simulink model "dynamic_model_dab_battery"  (R2022b)
settings: Solver=VariableStepAuto  StartTime=0.0  StopTime=5e-2  RelTol=1e-3
undefined symbols (not defined in the file): Ion, Lithium
libraries: spsMosfetLib x8, spsSeriesRLCBranchLib x6, spsEdgeDetectorLib x4, spsCurrentMeasurementLib x3, spsDiscreteVariableTimeDelayLib x2, spsBatteryLib x1, spsDCVoltageSourceLib x1, spsMultimeterLib x1, spsStairGeneratorLib x1, slpidlib x1, spsLinearTransformerLib x1, spsVoltageMeasurementLib x1
settings Model: Creator=srikr  LastModifiedBy=srikri

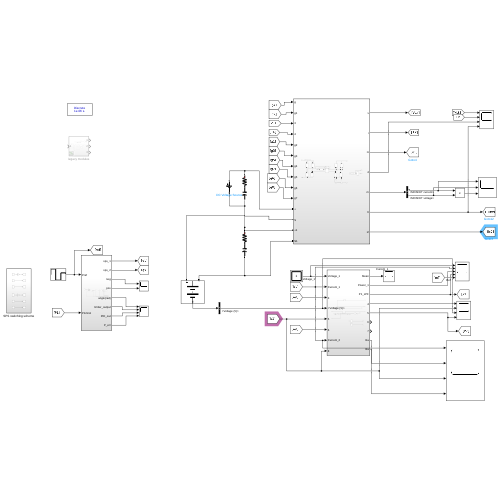
[thumbnail: Simulink's stored preview of the top-level diagram]
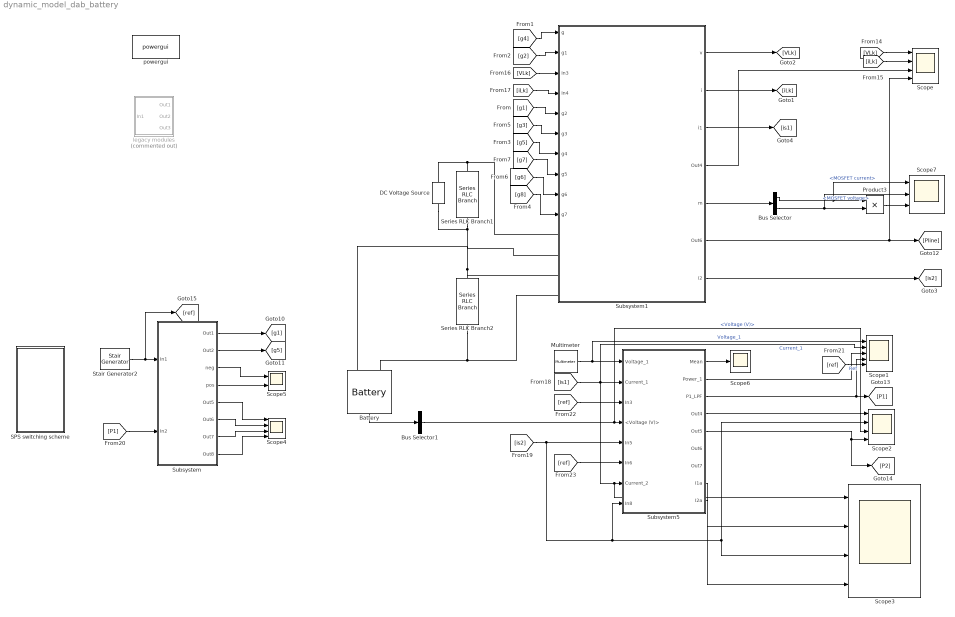
== system dynamic_model_dab_battery ==
  Battery : spsBatteryLib/Battery  BatType=Lithium-Ion  ShowTempParam=off  ThermalPreset=no  ShowAgeParam=off  NomV=96  NomQ=150  SOC=100  Batt_Tr=30  PresetModel=on  MaxQ=150  MinV=72  FullV=111.7428  Dis_rate=65.2174  R=0.0064  Normal_OP=135.6522  expZone="[103.717      7.369565]"  current=[6.5 13 32.5]  Units=Time  Tci=20  NomT=20  T2=-30  MaxQ2=4.8  FullV2=7.1  Normal_OP2=5.655  expZone2="[6.58           1]"  Rca=0.6  ti=2000  Dp=0  Neq0=0  Tsim=1e6  Ta1=25  Qeol=5.4*0.9  Reol=0.013333*1.2  Char_age=[2.3478, 3]  Dis_age=[2.3478, 10]  N1=1500  N2=10500  N3=1000  N4=1400  Ta2=45  N5=950
  Bus Selector : BusSelector  OutputSignals=MOSFET current,MOSFET voltage
  Bus Selector1 : BusSelector  OutputSignals=Voltage (V)
  DC Voltage Source : spsDCVoltageSourceLib/DC Voltage Source  Amplitude=120  Measurements=Voltage
  Multimeter : spsMultimeterLib/Multimeter  L=10  sel=4  yselected={}  Gain=1  OutputType=Complex  PlotAtSimulationStop=off  PhasorSimulation=off
  Product3 : Product
  SPS switching scheme : Subsystem
  Scope{,2..4} (4 alike) : Scope  NumInputPorts=4
  Scope1 : Scope  NumInputPorts=5
  Scope5 : Scope  NumInputPorts=2
  Scope6 : Scope
  Scope7 : Scope  NumInputPorts=3
  Series RLC Branch1 : spsSeriesRLCBranchLib/Series RLC Branch  LConnTagsString=__new0  RConnTagsString=__new0  BranchType=RC  Resistance=1e-9  Inductance=1e-3  SetiL0=off  InitialCurrent=0  Capacitance=1000e-6  Setx0=off  InitialVoltage=0  Measurements=None
  Series RLC Branch2 : spsSeriesRLCBranchLib/Series RLC Branch  LConnTagsString=__new0  RConnTagsString=__new0  BranchType=RC  Resistance=1e-9  Inductance=1e-3  SetiL0=off  InitialCurrent=0  Capacitance=1000e-6  Setx0=off  InitialVoltage=0  Measurements=None
  Stair Generator2 : spsStairGeneratorLib/Stair Generator  t=[0:.25:1]*4e-2  e=[0e3,3.5e3,-3.5e3,1e3,0.5e3]  Ts=0
  Subsystem : Subsystem
  Subsystem1 : Subsystem
  Subsystem5 : Subsystem
  legacy modules : Subsystem  Commented=on
  powergui : spspowerguiLib/powergui  Priority=1  SimulationMode=Discrete  SampleTime=1e-6  frequency=60  Iterations=50  frequencyindice=0  Pbase=100e6  ErrMax=1e-4  UnitsV=kV  UnitsW=MW  buscounter=0  FunctionMessages=off  echomessages=off  EnableUseOfTLC=off  CurrentSourceSwitches=off  DisableSnubberDevices=off  DisableRonSwitches=off  DisableVfSwitches=off  DisplayEquations=off  AutomaticDiscreteSolvers=off  SolverType=Tustin/Backward Euler (TBE)  Interpol=off  ExternalGateDelay=off  methode=off  Ts=100  x0status=blocks  SPID=on  SwTol=0  HookPort=off  NonlinearTolerance=1e-4  nMaxIteration=100  ContinueOnMaxIteration=off  RestoreLinks=warning  ResistiveCurrentMeasurement=off  Frange=[0:2:500]  Ylog=off  Xlog=on  ShowGrid=off  save=off  variable=ZData  structure=0  ZoomFFT=off  StartTime=0.0  cycles=1  DisplayStyle=1  fundamental=60  FreqAxis=off  MaxFrequency=1000  frequencyindicesteady=1  RmsSteady=1  display=off
  wires:
  [VLk] -> Scope/1
  [iLk] -> Scope/2
  Multimeter/1 -> Scope1/1, Subsystem5/1(Voltage_1)  "Voltage_1"
  [is1] -> Scope1/2, Scope3/1, Subsystem5/7(Current_2), Subsystem5/2(Current_1)  "Current_1"
  [is2] -> Scope2/2, Scope3/3, Subsystem5/8(In8), Subsystem5/5(In5)
  Bus Selector1/1 -> Scope2/1, Subsystem5/4(<Voltage (V)>)  "<Voltage (V)>"
  Stair Generator2/1 -> [ref], Subsystem/1(In1)
  Bus Selector/1 -> Scope7/1, Product3/1  "<MOSFET current>"
  Bus Selector/2 -> Scope7/2, Product3/2  "<MOSFET voltage>"
  Product3/1 -> Scope7/3
  [ref] -> Scope1/5  "Ref"
  Battery/1 -> Bus Selector1/1
  [P1] -> Subsystem/2(In2)
  Subsystem/1(Out1) -> [g1]
  Subsystem/2(Out2) -> [g5]
  Subsystem/3(neg) -> Scope5/1
  Subsystem/4(pos) -> Scope5/2
  Subsystem/5(Out5) -> Scope4/1
  Subsystem/6(Out6) -> Scope4/2
  Subsystem/7(Out7) -> Scope4/3
  Subsystem/8(Out8) -> Scope4/4
  Subsystem5/5(Out5) -> [P2], Scope2/4
  Subsystem5/3(P1_LPF) -> [P1], Scope1/4
  [ref] -> Subsystem5/3(In3)
  [ref] -> Subsystem5/6(In6)
  Subsystem5/1(Mean) -> Scope6/1
  Subsystem5/2(Power_1) -> Scope1/3
  Subsystem5/4(Out4) -> Scope2/3
  Subsystem5/8(I1a) -> Scope3/2
  Subsystem5/9(I2a) -> Scope3/4
  Subsystem1/6(Out6) -> [Pline], Scope/4
  [g4] -> Subsystem1/1(g)
  [g2] -> Subsystem1/2(g1)
  [VLk] -> Subsystem1/3(In3)
  [iLk] -> Subsystem1/4(In4)
  [g1] -> Subsystem1/5(g2)
  [g3] -> Subsystem1/6(g3)
  [g5] -> Subsystem1/7(g4)
  [g7] -> Subsystem1/8(g5)
  [g6] -> Subsystem1/9(g6)
  [g8] -> Subsystem1/10(g7)
  Subsystem1/1(v) -> [VLk]
  Subsystem1/2(i) -> [iLk]
  Subsystem1/3(i1) -> [is1]
  Subsystem1/4(Out4) -> Scope/3
  Subsystem1/5(m) -> Bus Selector/1
  Subsystem1/7(i2) -> [is2]
  connections:
  Series RLC Branch1/RConn1 -- DC Voltage Source/LConn1 -- Subsystem1/LConn2
  Series RLC Branch2/RConn1 -- Battery/LConn2 -- Subsystem1/LConn4
  Series RLC Branch2/LConn1 -- Battery/LConn1 -- Subsystem1/LConn3
  DC Voltage Source/RConn1 -- Subsystem1/LConn1 -- Series RLC Branch1/LConn1

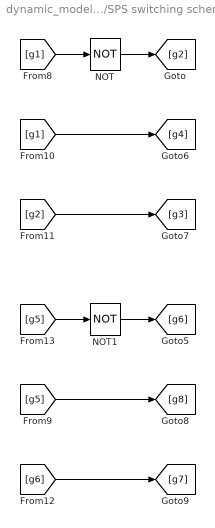
== system dynamic_model_dab_battery/SPS switching scheme ==
  NOT : Logic  Operator=NOT  IconShape=distinctive  AllPortsSameDT=off  OutDataTypeStr=boolean
  NOT1 : Logic  Operator=NOT  IconShape=distinctive  AllPortsSameDT=off  OutDataTypeStr=boolean
  wires:
  [g1] -> [g4]
  [g2] -> [g3]
  [g5] -> NOT1/1
  [g6] -> [g7]
  NOT1/1 -> [g6]
  [g5] -> [g8]
  NOT/1 -> [g2]
  [g1] -> NOT/1

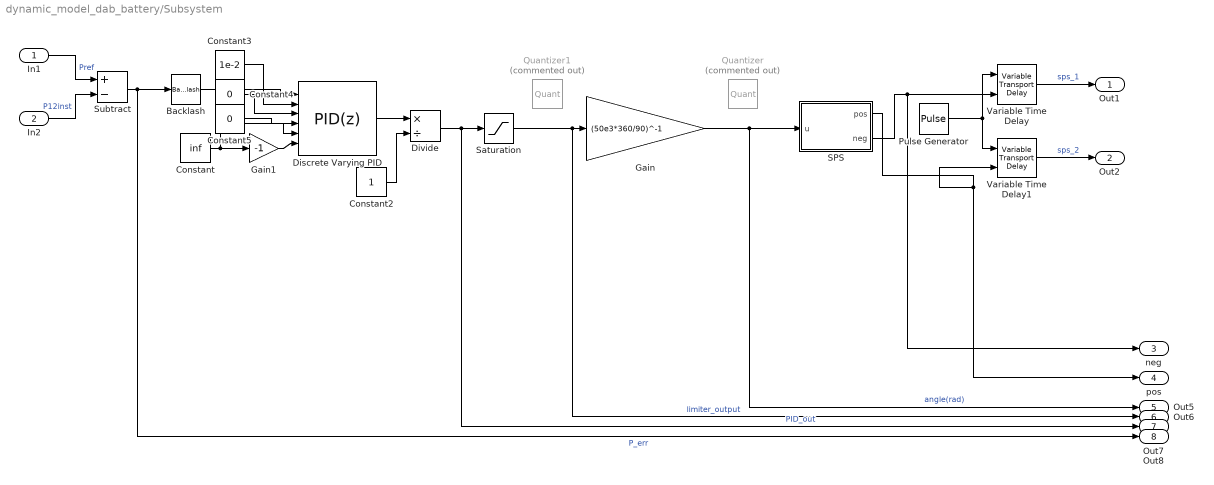
== system dynamic_model_dab_battery/Subsystem ==
  In1 : Inport
  In2 : Inport  Port=2
  Backlash : Backlash  BacklashWidth=0
  Constant : Constant  Value=inf
  Constant2 : Constant
  Constant3 : Constant  Value=1e-2
  Constant4 : Constant  Value=0
  Constant5 : Constant  Value=0
  Discrete Varying PID : slpidlib/PID Controller  Controller=PID  Form=Parallel  TimeDomain=Discrete-time  UseExternalTs=off  SampleTime=-1  IntegratorMethod=Forward Euler  FilterMethod=Forward Euler  ControllerParametersSource=external  P=1  I=1  UseKiTs=off  D=0  N=100  UseFilter=off  TunerSelectOption=Transfer Function Based (PID Tuner App)  InitialConditionSource=internal  InitialConditionForIntegrator=0  InitialConditionForFilter=0  DifferentiatorICPrevScaledInput=0  ExternalReset=none  TrackingMode=off  Kt=1  LimitOutput=on  SatLimitsSource=external  UpperSaturationLimit=inf  LowerSaturationLimit=-inf  LinearizeAsGain=on  AntiWindupMode=none  Kb=1  LimitIntegrator=off  UpperIntegratorSaturationLimit=inf  LowerIntegratorSaturationLimit=-inf  POutMin=[]  POutMax=[]  IOutMin=[]  IOutMax=[]  DOutMin=[]  DOutMax=[]  NOutMin=[]  NOutMax=[]  SumOutMin=[]  SumOutMax=[]  SaturationOutMin=[]  SaturationOutMax=[]  PParamMin=[]  PParamMax=[]  IParamMin=[]  IParamMax=[]  DParamMin=[]  DParamMax=[]  NParamMin=[]  NParamMax=[]  KbParamMin=[]  KbParamMax=[]  KtParamMin=[]  KtParamMax=[]  KbOutMin=[]  KbOutMax=[]  KtOutMin=[]  KtOutMax=[]  IntegratorOutMin=[]  IntegratorOutMax=[]  FilterOutMin=[]  FilterOutMax=[]  SumI1OutMin=[]  SumI1OutMax=[]  SumI2OutMin=[]  SumI2OutMax=[]  SumI3OutMin=[]  SumI3OutMax=[]  SumI4OutMin=[]  SumI4OutMax=[]  SumDOutMin=[]  SumDOutMax=[]  DifferentiatorOutMin=[]  DifferentiatorOutMax=[]  FilterDiffOutCoefMin=[]  FilterDiffOutCoefMax=[]  ReciprocalOutMin=[]  ReciprocalOutMax=[]  SumDenOutMin=[]  SumDenOutMax=[]  SumNumOutMin=[]  SumNumOutMax=[]  DivideOutMin=[]  DivideOutMax=[]  UdiffTsProdOutMin=[]  UdiffTsProdOutMax=[]  NTsProdOutMin=[]  NTsProdOutMax=[]  UintegralTsProdOutMin=[]  UintegralTsProdOutMax=[]  UngainTsProdOutMin=[]  UngainTsProdOutMax=[]  ClampingZeroOutDataTypeStr=Inherit: Inherit via back propagation  ClampingZeroOutMin=[]  ClampingZeroOutMax=[]  FilterDenConstantOutDataTypeStr=Inherit: Inherit via back propagation  FilterDenConstantOutMin=[]  FilterDenConstantOutMax=[]  PCopyOutDataTypeStr=Inherit: Inherit via back propagation  PCopyOutMin=[]  PCopyOutMax=[]  NCopyOutDataTypeStr=Inherit: Inherit via back propagation  NCopyOutMin=[]  NCopyOutMax=[]  IntegratorContinuousStateAttributes=''  IntegratorStateMustResolveToSignalObject=off  IntegratorRTWStateStorageClass=Auto  FilterContinuousStateAttributes=''  FilterStateMustResolveToSignalObject=off  FilterRTWStateStorageClass=Auto  ParallelPVariant=ExternalParameters  IdealPVariant=Disabled  IVariant=ExternalParameters  DVariant=ExternalParameters  IntegratorVariant=Discrete  SatVariant=External  AWVariant=Passthrough  PCopyVariant=Disabled  TRVariant=Disabled  FdbkBlocksVariant=Forward  IdealPFdbkVariant=Disabled  SatFdbkVariant=Disabled  DerivativeFilterVariant=Differentiator  NVariant=Passthrough  NCopyVariant=Disabled_SignalSpec  FilterICVariant=InternalICsDifferentiator  IntegratorICVariant=InternalICs  ExternalResetVariant=Disabled  TRSumVariant=Passthrough  SumFdbkVariant=Disabled  SumVariant=Sum_PID  TsampFilterVariant=InternalTs  TsampNgainVariant=Passthrough  TsampIntegralVariant=Passthrough  ExternalSaturationOutDataTypeStr=Inherit: Same as second input
      settings: LibrarySourceBlock=cstblocks/Linear Parameter Varying/Discrete Varying PID
  Divide : Product  Inputs=*/
  Gain : Gain  Gain=(50e3*360/90)^-1
  Gain1 : Gain  Gain=-1
  Pulse Generator : DiscretePulseGenerator  PulseType=Time based  Period=1/50e3  PulseWidth=50
  Quantizer : Quantizer  Commented=on  QuantizationInterval=1e-5
  Quantizer1 : Quantizer  Commented=on  QuantizationInterval=1e-2
  SPS : MATLAB Function  TreatAsAtomicUnit=on
  Saturation : Saturate  UpperLimit=1  LowerLimit=-1
  Subtract : Sum  Inputs=+-
  Variable Time Delay : VariableTransportDelay  MaximumDelay=10
  Variable Time Delay1 : VariableTransportDelay  MaximumDelay=10
  Out1 : Outport
  Out2 : Outport  Port=2
  neg : Outport  Port=3
  pos : Outport  Port=4
  Out5 : Outport  Port=5
  Out6 : Outport  Port=6
  Out7 : Outport  Port=7
  Out8 : Outport  Port=8
  wires:
  Backlash/1 -> Discrete Varying PID/1
  Constant2/1 -> Divide/2
  Constant4/1 -> Discrete Varying PID/3
  In1/1 -> Subtract/1  "Pref"
  Variable Time Delay/1 -> Out1/1  "sps_1"
  Saturation/1 -> Out6/1, Gain/1  "limiter_output"
  SPS/1(pos) -> pos/1, Variable Time Delay1/2
  SPS/2(neg) -> neg/1, Variable Time Delay/2
  Variable Time Delay1/1 -> Out2/1  "sps_2"
  In2/1 -> Subtract/2  "P12inst"
  Constant/1 -> Discrete Varying PID/5, Gain1/1
  Constant5/1 -> Discrete Varying PID/4
  Pulse Generator/1 -> Variable Time Delay1/1, Variable Time Delay/1
  Constant3/1 -> Discrete Varying PID/2
  Divide/1 -> Out7/1, Saturation/1  "PID_out"
  Discrete Varying PID/1 -> Divide/1
  Subtract/1 -> Out8/1, Backlash/1  "P_err"
  Gain1/1 -> Discrete Varying PID/6
  Gain/1 -> Out5/1, SPS/1(u)  "angle(rad)"

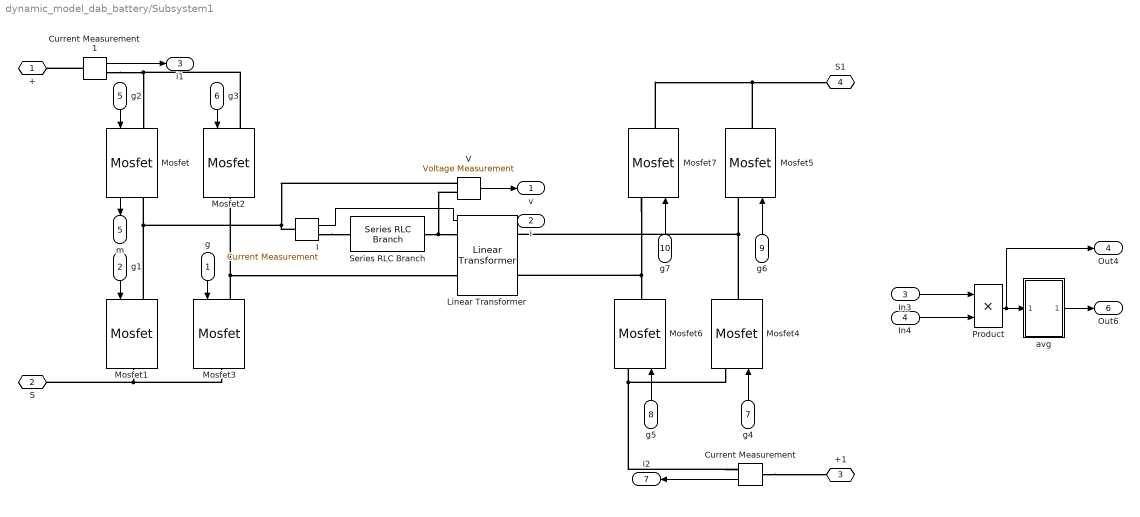
== system dynamic_model_dab_battery/Subsystem1 ==
  g : Inport
  g1 : Inport  Port=2
  In3 : Inport  Port=3
  In4 : Inport  Port=4
  g2 : Inport  Port=5
  g3 : Inport  Port=6
  g4 : Inport  Port=7
  g5 : Inport  Port=8
  g6 : Inport  Port=9
  g7 : Inport  Port=10
  Current Measurement : spsCurrentMeasurementLib/Current Measurement  PhasorSimulation=off  OutputType=Complex  PSBequivalent=0
  Current Measurement1 : spsCurrentMeasurementLib/Current Measurement  PhasorSimulation=off  OutputType=Complex  PSBequivalent=0
  I : spsCurrentMeasurementLib/Current Measurement  PhasorSimulation=off  OutputType=Complex  PSBequivalent=0
  Linear Transformer : spsLinearTransformerLib/Linear Transformer  UNITS=SI  NominalPower=[ 3.5e3 50e3 ]  winding1=[120 0 0]  winding2=[96 0 0]  ThreeWindings=off  winding3=[3.15e+05 0.7938 0.084225]  RmLm=[10e6 2e-3]  Measurements=All voltages and currents  DataType=on
  Mosfet : spsMosfetLib/Mosfet  Ron=0.1  Lon=0  Rd=0.01  Vfd=0  IC=0  Rs=1e6  Cs=inf  Measurements=on
  Mosfet1 : spsMosfetLib/Mosfet  Ron=0.1  Lon=0  Rd=0.01  Vfd=0  IC=0  Rs=inf  Cs=inf  Measurements=off
  Mosfet{2..7} (6 alike) : spsMosfetLib/Mosfet  Ron=0.1  Lon=0  Rd=0.01  Vfd=0  IC=0  Rs=1e6  Cs=inf  Measurements=off
  Product : Product
  Series RLC Branch : spsSeriesRLCBranchLib/Series RLC Branch  LConnTagsString=__new0  RConnTagsString=__new0  BranchType=L  Resistance=1  Inductance=15e-6  SetiL0=off  InitialCurrent=0  Capacitance=1e-6  Setx0=off  InitialVoltage=0  Measurements=Branch voltage and current
  V : spsVoltageMeasurementLib/Voltage Measurement  PhasorSimulation=off  OutputType=Complex  PSBequivalent=0
  avg : Subsystem
  + : PMIOPort  Side=Left
  S : PMIOPort  Port=2  Side=Left
  +1 : PMIOPort  Port=3  Side=Left
  S1 : PMIOPort  Port=4  Side=Left
  v : Outport
  i : Outport  Port=2
  i1 : Outport  Port=3
  Out4 : Outport  Port=4
  m : Outport  Port=5
  Out6 : Outport  Port=6
  i2 : Outport  Port=7
  wires:
  V/1 -> v/1
  g5/1 -> Mosfet6/1
  In3/1 -> Product/1
  g6/1 -> Mosfet5/1
  In4/1 -> Product/2
  Mosfet/1 -> m/1
  g2/1 -> Mosfet/1
  g4/1 -> Mosfet4/1
  I/1 -> i/1
  Current Measurement1/1 -> i1/1
  Current Measurement/1 -> i2/1
  g1/1 -> Mosfet1/1
  g/1 -> Mosfet3/1
  avg/1(Out1) -> Out6/1
  g3/1 -> Mosfet2/1
  g7/1 -> Mosfet7/1
  Product/1 -> Out4/1, avg/1(In1)
  connections:
  Mosfet7/LConn1 -- Mosfet6/RConn1 -- Linear Transformer/RConn2
  Current Measurement1/RConn1 -- Mosfet/LConn1 -- Mosfet2/LConn1
  Series RLC Branch/RConn1 -- V/LConn2 -- Linear Transformer/LConn1
  Current Measurement/LConn1 -- +1/RConn1
  Current Measurement/RConn1 -- Mosfet4/LConn1 -- Mosfet6/LConn1
  Mosfet4/RConn1 -- Mosfet5/LConn1 -- Linear Transformer/RConn1
  Current Measurement1/LConn1 -- +/RConn1
  Mosfet3/RConn1 -- S/RConn1 -- Mosfet1/RConn1
  I/LConn1 -- V/LConn1 -- Mosfet1/LConn1 -- Mosfet/RConn1
  I/RConn1 -- Series RLC Branch/LConn1
  Mosfet7/RConn1 -- Mosfet5/RConn1 -- S1/RConn1
  Mosfet3/LConn1 -- Linear Transformer/LConn2 -- Mosfet2/RConn1

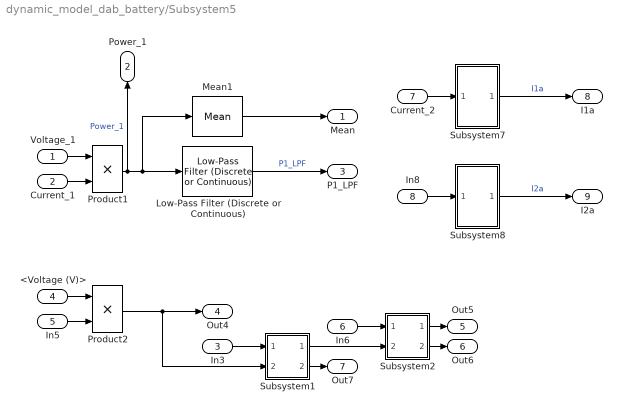
== system dynamic_model_dab_battery/Subsystem5 ==
  Voltage_1 : Inport
  Current_1 : Inport  Port=2
  In3 : Inport  Port=3
  <Voltage (V)> : Inport  Port=4
  In5 : Inport  Port=5
  In6 : Inport  Port=6
  Current_2 : Inport  Port=7
  In8 : Inport  Port=8
  Low-Pass Filter (Discrete or Continuous) : eeGeneralControl/Low-Pass Filter (Discrete or Continuous)  K=1  T=1e-3  B=inf  A=-inf  init_option=Specify as parameter  x0=0  Ts=-1
  Mean1 : spsMeanLib/Mean  Freq=25e3  Vinit=0  Ts=0
  Product1 : Product
  Product2 : Product
  Subsystem1 : Subsystem
  Subsystem2 : Subsystem
  Subsystem7 : Subsystem
  Subsystem8 : Subsystem
  Mean : Outport
  Power_1 : Outport  Port=2
  P1_LPF : Outport  Port=3
  Out4 : Outport  Port=4
  Out5 : Outport  Port=5
  Out6 : Outport  Port=6
  Out7 : Outport  Port=7
  I1a : Outport  Port=8
  I2a : Outport  Port=9
  wires:
  Current_2/1 -> Subsystem7/1(In1)
  Subsystem7/1(Out1) -> I1a/1  "I1a"
  Subsystem8/1(Out1) -> I2a/1  "I2a"
  Current_1/1 -> Product1/2
  Low-Pass Filter (Discrete or Continuous)/1 -> P1_LPF/1  "P1_LPF"
  In8/1 -> Subsystem8/1(In1)
  Mean1/1 -> Mean/1
  Product2/1 -> Out4/1, Subsystem1/2(In2)
  Product1/1 -> Low-Pass Filter (Discrete or Continuous)/1, Mean1/1, Power_1/1  "Power_1"
  In6/1 -> Subsystem2/1(In1)
  <Voltage (V)>/1 -> Product2/1
  In3/1 -> Subsystem1/1(In1)
  Subsystem2/2(Out2) -> Out6/1
  Voltage_1/1 -> Product1/1
  In5/1 -> Product2/2
  Subsystem1/1(Out1) -> Subsystem2/2(In2)
  Subsystem2/1(Out1) -> Out5/1
  Subsystem1/2(Out2) -> Out7/1

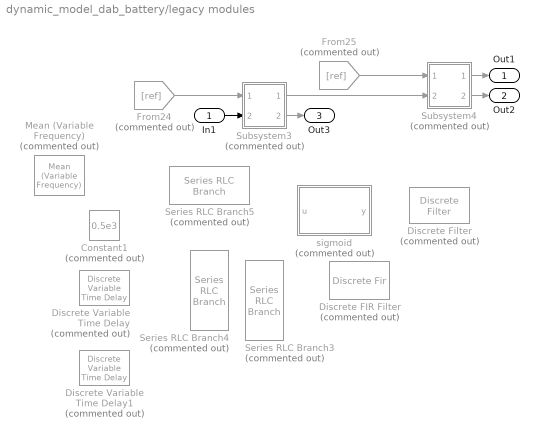
== system dynamic_model_dab_battery/legacy modules ==
  In1 : Inport
  Constant1 : Constant  Commented=on  Value=0.5e3
  Discrete FIR Filter : DiscreteFir  Commented=on
  Discrete Filter : DiscreteFilter  Commented=on
  Discrete Variable Time Delay : spsDiscreteVariableTimeDelayLib/Discrete Variable Time Delay  Commented=on  MaxDelay=1  InitialValue=0  Ts=1e-4  DFT=on
      settings: LibrarySourceBlock=|
      | sps_lib/Control/Discrete Variable
      | Time Delay
  Discrete Variable Time Delay1 : spsDiscreteVariableTimeDelayLib/Discrete Variable Time Delay  Commented=on  MaxDelay=1  InitialValue=0  Ts=1e-4  DFT=on
      settings: LibrarySourceBlock=|
      | sps_lib/Control/Discrete Variable
      | Time Delay
  From24 : From  Commented=on  GotoTag=ref
  From25 : From  Commented=on  GotoTag=ref
  Mean (Variable Frequency) : spsMeanVariableFrequencyLib/Mean (Variable Frequency)  Commented=on  Finit=60  Fmin=45  Vinit=0  Ts=0
      settings: LibrarySourceBlock=|
      | sps_lib/Sensors and Measurements/Mean
      | (Variable Frequency)
  Series RLC Branch3 : spsSeriesRLCBranchLib/Series RLC Branch  Commented=on  LConnTagsString=__new0  RConnTagsString=__new0  BranchType=L  Resistance=1  Inductance=1e-6/(1.25^2)  SetiL0=off  InitialCurrent=0  Capacitance=1e-6  Setx0=off  InitialVoltage=0  Measurements=Branch voltage and current
  Series RLC Branch4 : spsSeriesRLCBranchLib/Series RLC Branch  Commented=on  LConnTagsString=__new0  RConnTagsString=__new0  BranchType=C  Resistance=1  Inductance=14e-6  SetiL0=off  InitialCurrent=0  Capacitance=10e-6*(1.25^2)  Setx0=off  InitialVoltage=0  Measurements=Branch voltage and current
  Series RLC Branch5 : spsSeriesRLCBranchLib/Series RLC Branch  Commented=on  LConnTagsString=__new0  RConnTagsString=__new0  BranchType=C  Resistance=1  Inductance=14e-6  SetiL0=off  InitialCurrent=0  Capacitance=10e-6  Setx0=off  InitialVoltage=0  Measurements=Branch voltage and current
  Subsystem3 : Subsystem  Commented=on
  Subsystem4 : Subsystem  Commented=on
  sigmoid : MATLAB Function  Commented=on  TreatAsAtomicUnit=on
  Out1 : Outport
  Out2 : Outport  Port=2
  Out3 : Outport  Port=3
  wires:
  Subsystem3/1(Out1) -> Subsystem4/2(In2)
  From25/1 -> Subsystem4/1(In1)
  From24/1 -> Subsystem3/1(In1)
  In1/1 -> Subsystem3/2(In2)
  Subsystem4/2(Out2) -> Out2/1
  Subsystem4/1(Out1) -> Out1/1
  Subsystem3/2(Out2) -> Out3/1

== system dynamic_model_dab_battery/Subsystem1/avg ==
  In1 : Inport
  Clock : Clock
  Divide : Product  Inputs=*/
  Integrator : Integrator
  Out1 : Outport
  wires:
  Divide/1 -> Out1/1
  Clock/1 -> Divide/2
  Integrator/1 -> Divide/1
  In1/1 -> Integrator/1

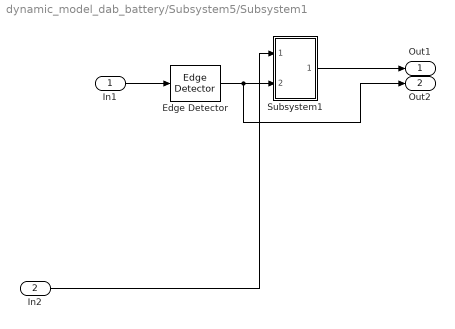
== system dynamic_model_dab_battery/Subsystem5/Subsystem1 ==
  In1 : Inport
  In2 : Inport  Port=2
  Edge Detector : spsEdgeDetectorLib/Edge Detector  model=Either  ic=0  Ts=0
      settings: LibrarySourceBlock=sps_lib/Control/Edge Detector
  Subsystem1 : Subsystem
  Out1 : Outport
  Out2 : Outport  Port=2
  wires:
  Edge Detector/1 -> Out2/1, Subsystem1/2(Input)
  Subsystem1/1(Out1) -> Out1/1
  In1/1 -> Edge Detector/1
  In2/1 -> Subsystem1/1(In1)

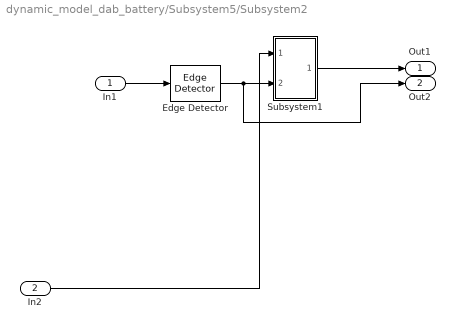
== system dynamic_model_dab_battery/Subsystem5/Subsystem2 ==
  In1 : Inport
  In2 : Inport  Port=2
  Edge Detector : spsEdgeDetectorLib/Edge Detector  model=Either  ic=0  Ts=0
      settings: LibrarySourceBlock=sps_lib/Control/Edge Detector
  Subsystem1 : Subsystem
  Out1 : Outport
  Out2 : Outport  Port=2
  wires:
  Edge Detector/1 -> Out2/1, Subsystem1/2(Input)
  Subsystem1/1(Out1) -> Out1/1
  In1/1 -> Edge Detector/1
  In2/1 -> Subsystem1/1(In1)

== system dynamic_model_dab_battery/Subsystem5/Subsystem7 ==
  In1 : Inport
  Clock : Clock
  Divide : Product  Inputs=*/
  Integrator : Integrator
  Switch : Switch  Criteria=u2 > Threshold  SaturateOnIntegerOverflow=off  InputSameDT=off
  Out1 : Outport
  wires:
  Divide/1 -> Switch/1
  Integrator/1 -> Switch/3, Divide/1
  Clock/1 -> Switch/2, Divide/2
  In1/1 -> Integrator/1
  Switch/1 -> Out1/1

== system dynamic_model_dab_battery/Subsystem5/Subsystem8 ==
  In1 : Inport
  Clock : Clock
  Divide : Product  Inputs=*/
  Integrator : Integrator
  Switch : Switch  Criteria=u2 > Threshold  SaturateOnIntegerOverflow=off  InputSameDT=off
  Out1 : Outport
  wires:
  Divide/1 -> Switch/1
  Integrator/1 -> Switch/3, Divide/1
  Clock/1 -> Switch/2, Divide/2
  In1/1 -> Integrator/1
  Switch/1 -> Out1/1

== system dynamic_model_dab_battery/legacy modules/Subsystem3 ==
  In1 : Inport
  In2 : Inport  Port=2
  Edge Detector : spsEdgeDetectorLib/Edge Detector  model=Either  ic=0  Ts=0
      settings: LibrarySourceBlock=sps_lib/Control/Edge Detector
  Subsystem1 : Subsystem
  Out1 : Outport
  Out2 : Outport  Port=2
  wires:
  Edge Detector/1 -> Out2/1, Subsystem1/2(Input)
  Subsystem1/1(Out1) -> Out1/1
  In1/1 -> Edge Detector/1
  In2/1 -> Subsystem1/1(In1)

== system dynamic_model_dab_battery/legacy modules/Subsystem4 ==
  In1 : Inport
  In2 : Inport  Port=2
  Edge Detector : spsEdgeDetectorLib/Edge Detector  model=Either  ic=0  Ts=0
      settings: LibrarySourceBlock=sps_lib/Control/Edge Detector
  Subsystem1 : Subsystem
  Out1 : Outport
  Out2 : Outport  Port=2
  wires:
  Edge Detector/1 -> Out2/1, Subsystem1/2(Input)
  Subsystem1/1(Out1) -> Out1/1
  In1/1 -> Edge Detector/1
  In2/1 -> Subsystem1/1(In1)

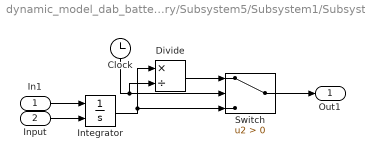
== system dynamic_model_dab_battery/Subsystem5/Subsystem1/Subsystem1 ==
  In1 : Inport
  Input : Inport  Port=2
  Clock : Clock
  Divide : Product  Inputs=*/
  Integrator : Integrator  ExternalReset=rising  LimitOutput=on  IgnoreLimit=on
  Switch : Switch  Criteria=u2 > Threshold  SaturateOnIntegerOverflow=off  InputSameDT=off
  Out1 : Outport
  wires:
  Divide/1 -> Switch/1
  Integrator/1 -> Switch/3, Divide/1
  Clock/1 -> Switch/2, Divide/2
  In1/1 -> Integrator/1
  Switch/1 -> Out1/1
  Input/1 -> Integrator/2

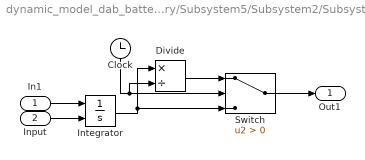
== system dynamic_model_dab_battery/Subsystem5/Subsystem2/Subsystem1 ==
  In1 : Inport
  Input : Inport  Port=2
  Clock : Clock
  Divide : Product  Inputs=*/
  Integrator : Integrator  ExternalReset=rising  LimitOutput=on  IgnoreLimit=on
  Switch : Switch  Criteria=u2 > Threshold  SaturateOnIntegerOverflow=off  InputSameDT=off
  Out1 : Outport
  wires:
  Divide/1 -> Switch/1
  Integrator/1 -> Switch/3, Divide/1
  Clock/1 -> Switch/2, Divide/2
  In1/1 -> Integrator/1
  Switch/1 -> Out1/1
  Input/1 -> Integrator/2

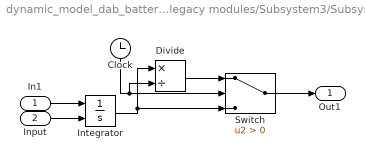
== system dynamic_model_dab_battery/legacy modules/Subsystem3/Subsystem1 ==
  In1 : Inport
  Input : Inport  Port=2
  Clock : Clock
  Divide : Product  Inputs=*/
  Integrator : Integrator  ExternalReset=rising  LimitOutput=on  IgnoreLimit=on
  Switch : Switch  Criteria=u2 > Threshold  SaturateOnIntegerOverflow=off  InputSameDT=off
  Out1 : Outport
  wires:
  Divide/1 -> Switch/1
  Integrator/1 -> Switch/3, Divide/1
  Clock/1 -> Switch/2, Divide/2
  In1/1 -> Integrator/1
  Switch/1 -> Out1/1
  Input/1 -> Integrator/2

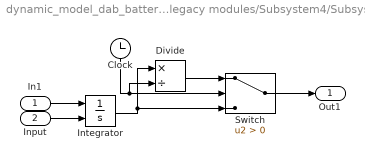
== system dynamic_model_dab_battery/legacy modules/Subsystem4/Subsystem1 ==
  In1 : Inport
  Input : Inport  Port=2
  Clock : Clock
  Divide : Product  Inputs=*/
  Integrator : Integrator  ExternalReset=rising  LimitOutput=on  IgnoreLimit=on
  Switch : Switch  Criteria=u2 > Threshold  SaturateOnIntegerOverflow=off  InputSameDT=off
  Out1 : Outport
  wires:
  Divide/1 -> Switch/1
  Integrator/1 -> Switch/3, Divide/1
  Clock/1 -> Switch/2, Divide/2
  In1/1 -> Integrator/1
  Switch/1 -> Out1/1
  Input/1 -> Integrator/2

== matlab function dynamic_model_dab_battery/legacy modules/sigmoid ==
  data: u input; y output
function y = fcn(u)

y = 1/(1 + exp(-u));

== matlab function dynamic_model_dab_battery/Subsystem/SPS ==
  data: u input; pos output; neg output
function [pos,neg] = fcn(u)

if u>=0
    pos = abs(u);
    neg = 0;
else
    neg = abs(u);
    pos = 0;
end
